simulink model "DIAGRAMADEBLOQUEPREGUNTA4"  (R2018b)
settings: Solver=VariableStepAuto  StartTime=0.0  StopTime=10.0  RelTol=1e-3
libraries: simulink x2
settings Model: Creator=Harold  LastModifiedBy=Harold

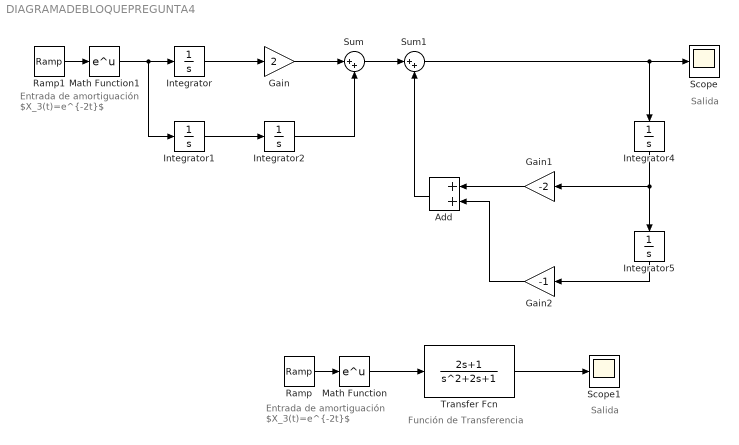
== system DIAGRAMADEBLOQUEPREGUNTA4 ==
  note: Función de Transferencia
  note: Entrada de amortiguación
      | $X_3(t)=e^{-2t}$
  note: Salida
  note: Salida
  note: Entrada de amortiguación
      | $X_3(t)=e^{-2t}$
  Add : Sum
  Gain : Gain  Gain=2
  Gain1 : Gain  Gain=-2
  Gain2 : Gain  Gain=-1
  Integrator{,1..2,4..5} (5 alike) : Integrator
  Math Function : Math  SaturateOnIntegerOverflow=on
  Math Function1 : Math  SaturateOnIntegerOverflow=on
  Ramp : simulink/Sources/Ramp  slope=-2  start=0  InitialOutput=0
  Ramp1 : simulink/Sources/Ramp  slope=-2  start=0  InitialOutput=0
  Scope : Scope
  Scope1 : Scope
  Sum : Sum  Inputs=|++
  Sum1 : Sum  Inputs=|++
  Transfer Fcn : TransferFcn  Numerator=[2 1]
  wires:
  Integrator1/1 -> Integrator2/1
  Integrator/1 -> Gain/1
  Gain/1 -> Sum/1
  Integrator2/1 -> Sum/2
  Integrator4/1 -> Integrator5/1, Gain1/1
  Integrator5/1 -> Gain2/1
  Sum/1 -> Sum1/1
  Add/1 -> Sum1/2
  Sum1/1 -> Scope/1, Integrator4/1
  Math Function1/1 -> Integrator1/1, Integrator/1
  Gain1/1 -> Add/1
  Gain2/1 -> Add/2
  Math Function/1 -> Transfer Fcn/1
  Transfer Fcn/1 -> Scope1/1
  Ramp/1 -> Math Function/1
  Ramp1/1 -> Math Function1/1
